simulink model "Citation"  (R2018a)
settings: Solver=ode5  StartTime=0.0  StopTime=500  FixedStep=0.01  RelTol=1e-3  EnableMultiTasking=on
InitFcn:
  | initcit
values from neighbouring files (symbols this model uses):
  aeroinit = [dp_ini;inicoef('CX0');inicoef('CXa');inicoef('CXa2');inicoef('CXq')     ;inicoef('CXde');inicoef('CY0');inicoef('CYB');inicoef('CYp');inicoef('CYr')     ;inicoef('CYda');inicoef('CYdr');inicoef('CZ0');inicoef('CZa');inicoef('CZq')     ;inicoef('CZde');inicoef('Cl0');inicoef('ClB');inicoef('Clp');inicoef('Clr')     ;inicoef('Clda');inicoef('Cldr');inicoef('Cm0');inicoef('Cma');inicoef('Cmq')     ; ...(+113 chars)    [initcit.m]
  h_l_old = zeros(6,sample_size)    [initcit.m]
  h_m_old = zeros(4,sample_size)    [initcit.m]
  h_n_old = zeros(6,sample_size)    [initcit.m]
  h_X_old = zeros(5,sample_size)    [initcit.m]
  h_Y_old = zeros(6,sample_size)    [initcit.m]
  h_Z_old = zeros(4,sample_size)    [initcit.m]
  I = [massinit(5),0, -massinit(8);0, massinit(6),0;-massinit(8),0, massinit(7)]    [initcit.m]
  p_l = [inicoef('Cl0');inicoef('ClB');inicoef('Clp');inicoef('Clr')     ;inicoef('Clda');inicoef('Cldr')].*ones(6,sample_size)    [initcit.m]
  p_m = [inicoef('Cm0');inicoef('Cma');inicoef('Cmq')     ;inicoef('Cmde')].*ones(4,sample_size)    [initcit.m]
  p_n = 0.71*ones(6,sample_size)    [initcit.m]
  p_X = [inicoef('CX0');inicoef('CXa');inicoef('CXa2');inicoef('CXq')     ;inicoef('CXde')].*ones(5,sample_size)    [initcit.m]
  p_Y = [inicoef('CY0');inicoef('CYB');inicoef('CYp');inicoef('CYr')     ;inicoef('CYda');inicoef('CYdr')].*ones(6,sample_size)    [initcit.m]
  p_Z = [inicoef('CZ0');inicoef('CZa');inicoef('CZq')     ;inicoef('CZde')].*ones(4,sample_size)    [initcit.m]
  Pcov_l = 10000*eye(6)    [initcit.m]
  Pcov_m = 10000*eye(4)    [initcit.m]
  Pcov_n = 10000*eye(6)    [initcit.m]
  Pcov_X = 10000*eye(5)    [initcit.m]
  Pcov_Y = 10000*eye(6)    [initcit.m]
  Pcov_Z = 10000*eye(4)    [initcit.m]
  T0 = 288.15    [rho_test.m]
  Vw915 = 0    [initcit.m]
  winddir = 45*(pi/180)    (= 0.785398163397)    [initcit.m]
  x0 = []    [cessnac550_3d_sfnc.m]    (also in sfunxyauto.m)
  y_l = zeros(1,sample_size)    [initcit.m]
  y_l_est_old = zeros(size(y_l))    [initcit.m]
  y_m = zeros(1,sample_size)    [initcit.m]
  y_m_est_old = zeros(size(y_m))    [initcit.m]
  y_n = zeros(1,sample_size)    [initcit.m]
  y_n_est_old = zeros(size(y_n))    [initcit.m]
  y_X = zeros(1,sample_size)    [initcit.m]
  y_X_est_old = zeros(size(y_X))    [initcit.m]
  y_Y = zeros(1,sample_size)    [initcit.m]
  y_Y_est_old = zeros(size(y_Y))    [initcit.m]
  y_Z = zeros(1,sample_size)    [initcit.m]
  y_Z_est_old = zeros(size(y_Z))    [initcit.m]
undefined symbols (not defined in the file or in its folder): chord, cv1, cv2, cv3, cv4, deltagmax1, deltagmax2, deltagmax3, deltagmax4, Deng, ealphag, ealphas, g0, hDME, hGS, kt1, kt2, kt3, lh, massinit, matbuaf, matdaf, matdam, matdbbf, matdeaf, matdgaf, matdqaf, matduaf, matdwaw, matedhr, mateif, matelhr, matemhr, matemv1, matemv2, matemve, matetam, mateuaf, matfaaf, matfaxl, matff, matibaf, matibb, matibmh, matipaf, matipmh, matiraf, matiuaf, matiwaf, matlaf, matlam, matleaf, matleam, matlgaf, matlqaf, matluaf, matmaaf, matmaam, matmaf, matmam ... (+75)
libraries: simulink x5, templibrary x3, vrlib x1
(part 6 of 6)

== matlab function Citation/Aerodynamic Parameter Estimation/CZ/MATLAB Function ==
  data: P_cov input; P_cov output; pk input; y_new input; hk_new input; y_old input; y_est_old input; h_old input; counter input; pk output; y_old output; y_est_old output; h_old output; forget input; counter output; y_est output; y_new output
function [P_cov, pk,y_old,y_est_old,h_old,counter,y_est,y_new] ...
    =LSQ(P_cov,pk,y_new,hk_new,y_old,y_est_old,h_old,counter,forget)
    lambda=forget;
    P=P_cov;
    p=pk(:,1);
    h=hk_new;
    y=y_new;
    Lk=P*h*(1/(h'*P*h+lambda));
    P=(eye(length(P))-Lk*h')*P*(1/lambda);
    
    p=p+Lk*(y-h'*p);   
    P_cov=P;   
    y_est=h'*p;
 
    
    %% Shift value history
    pk=shift(pk,p);
    y_est_old=(shift(y_est_old',y_est'))'; %this array is oriented vertically 
    h_old=shift(h_old,h);
    y_old=(shift(y_old',y_new'))';          %this array is oriented vertically 
    
    
    
    
    %shift array content right and insert new entry 
   
    function array = shift(array,insert)  

        for i=1:(size(array,2)-1)
             j=size(array,2)-i+1;
               array(:,j)=array(:,j-1);
        end
        array(:,1)=insert(:);

    end
%%
counter=counter+1;
end

== matlab function Citation/Aerodynamic Parameter Estimation/Cl/MATLAB Function ==
  data: P_cov input; P_cov output; pk input; y_new input; hk_new input; y_old input; y_est_old input; h_old input; counter input; pk output; y_old output; y_est_old output; h_old output; forget input; counter output; y_est output; y_new output
function [P_cov, pk,y_old,y_est_old,h_old,counter,y_est,y_new] ...
    =LSQ(P_cov,pk,y_new,hk_new,y_old,y_est_old,h_old,counter,forget)
    lambda=forget;
    P=P_cov;
    p=pk(:,1);
    h=hk_new;
    y=y_new;
    Lk=P*h*(1/(h'*P*h+lambda));
    P=(eye(length(P))-Lk*h')*P*(1/lambda);
    
    p=p+Lk*(y-h'*p);   
    P_cov=P;   
    y_est=h'*p;
 
    
    %% Shift value history
    pk=shift(pk,p);
    y_est_old=(shift(y_est_old',y_est'))'; %this array is oriented vertically 
    h_old=shift(h_old,h);
    y_old=(shift(y_old',y_new'))';          %this array is oriented vertically 
    
    
    
    
    %shift array content right and insert new entry 
   
    function array = shift(array,insert)  

        for i=1:(size(array,2)-1)
             j=size(array,2)-i+1;
               array(:,j)=array(:,j-1);
        end
        array(:,1)=insert(:);

    end
%%
counter=counter+1;
end

== matlab function Citation/Aerodynamic Parameter Estimation/Cm/MATLAB Function ==
  data: P_cov input; P_cov output; pk input; y_new input; hk_new input; y_old input; y_est_old input; h_old input; counter input; pk output; y_old output; y_est_old output; h_old output; forget input; counter output; y_est output; y_new output
function [P_cov, pk,y_old,y_est_old,h_old,counter,y_est,y_new] ...
    =LSQ(P_cov,pk,y_new,hk_new,y_old,y_est_old,h_old,counter,forget)
    lambda=forget;
    P=P_cov;
    p=pk(:,1);
    h=hk_new;
    y=y_new;
    Lk=P*h*(1/(h'*P*h+lambda));
    P=(eye(length(P))-Lk*h')*P*(1/lambda);
    
    p=p+Lk*(y-h'*p);   
    P_cov=P;   
    y_est=h'*p;
 
    
    %% Shift value history
    pk=shift(pk,p);
    y_est_old=(shift(y_est_old',y_est'))'; %this array is oriented vertically 
    h_old=shift(h_old,h);
    y_old=(shift(y_old',y_new'))';          %this array is oriented vertically 
    
    
    
    
    %shift array content right and insert new entry 
   
    function array = shift(array,insert)  

        for i=1:(size(array,2)-1)
             j=size(array,2)-i+1;
               array(:,j)=array(:,j-1);
        end
        array(:,1)=insert(:);

    end
%%
counter=counter+1;
end

== matlab function Citation/Aerodynamic Parameter Estimation/Cn/MATLAB Function ==
  data: P_cov input; P_cov output; pk input; y_new input; hk_new input; y_old input; y_est_old input; h_old input; counter input; pk output; y_old output; y_est_old output; h_old output; forget input; counter output; y_est output; y_new output
function [P_cov, pk,y_old,y_est_old,h_old,counter,y_est,y_new] ...
    =LSQ(P_cov,pk,y_new,hk_new,y_old,y_est_old,h_old,counter,forget)
    lambda=forget;
    P=P_cov;
    p=pk(:,1);
    h=hk_new;
    y=y_new;
    Lk=P*h*(1/(h'*P*h+lambda));
    P=(eye(length(P))-Lk*h')*P*(1/lambda);
    
    p=p+Lk*(y-h'*p);   
    P_cov=P;   
    y_est=h'*p;
 
    
    %% Shift value history
    pk=shift(pk,p);
    y_est_old=(shift(y_est_old',y_est'))'; %this array is oriented vertically 
    h_old=shift(h_old,h);
    y_old=(shift(y_old',y_new'))';          %this array is oriented vertically 
    
    
    
    
    %shift array content right and insert new entry 
   
    function array = shift(array,insert)  

        for i=1:(size(array,2)-1)
             j=size(array,2)-i+1;
               array(:,j)=array(:,j-1);
        end
        array(:,1)=insert(:);

    end
%%
counter=counter+1;
end

== matlab function Citation/Cessna Citation 500/Controllers/NDI rotational rate controller/b^-1 ==
  data: ve input; delta output; aerodat input; I parameter; chord parameter; span parameter; S parameter; mat_old output; mat_old input
function [delta, mat_old]  = fcn(ve,aerodat, I, chord, span, S,mat_old)
dp=aerodat(1); %dynamic pressure =0.5*rho*V^2*S
clda=aerodat(21);
cldr=aerodat(22);
cmde=aerodat(26);
cnda=aerodat(31);
cndr=aerodat(32);
mat=[span*clda, 0, span*cldr;
    0, chord*cmde, 0;
    span*cnda, 0, span*cndr];

if det(mat)==0 %take an older matrix if it is non-invertible
   mat=mat_old; 
else
    mat_old=mat;
end
amat=mat^(-1)*I;
delta=amat*(1/(dp))*ve;
dummy=1;

== matlab function Citation/Cessna Citation 500/Controllers/NDI rotational rate controller/a ==
  data: aerodat input; state input; y output; I parameter; span parameter; chord parameter
function y = fcn(aerodat,state, I, span, chord)
dp=aerodat(1);
p=state(1);
q=state(2);
r=state(3);
b=span;
c=chord;
V=state(4);
alpha=state(5);
beta=state(6);
Cl=aerodat(17:22);
Cm=aerodat(23:26);
Cn=aerodat(27:32);


Cla=Cl(1)+Cl(2)*beta+(Cl(3)*(p*b)/(2*V))+(Cl(4)*(r*b/(2*V)));
Cma=Cm(1)+Cm(2)*alpha+(Cm(3)*(q*c)/(2*V));
Cna=Cn(1)+Cn(2)*beta+(Cn(3)*(p*b)/(2*V))+(Cn(4)*(r*b/(2*V)));
term1=cross(state(1:3),I*state(1:3));
term2=dp*[b*Cla; c*Cma; b*Cna];
term3=term1-term2;
y=-1*(I^(-1)*term3);

== matlab function Citation/Aerodynamic Parameter Estimation/Statistics 2/Auto_correlation/autocorrelation ==
  data: delta input; PI_kgap output; kgap input; kgap_avg input; counter input; kgap_avg output; counter output
function [PI_kgap,kgap_avg,counter] = fcn(delta,kgap,kgap_avg,counter)

PI_kgap=(delta(1)*delta(1+kgap));
if counter>=1
    kgap_avg=kgap_avg+(PI_kgap/counter);
else
    kgap_avg=PI_kgap;
end

counter=counter+1;
end

== matlab function Citation/Aerodynamic Parameter Estimation/Statistics 2/moving average square ==
  data: delta input; av output
function av = fcn(delta)
av=0;
nav=length(delta);
k=nav;
for i=0:(nav-1)
    av=av+(delta(k-i))^2;
end
av=av/k;
end

== matlab function Citation/Aerodynamic Parameter Estimation/Statistics 2/variance/MATLAB Function ==
  data: delta input; var output; delta_avg input; counter input; delta_avg output; counter output; sigma_avg input; sigma_avg output
function [var,delta_avg,counter,sigma_avg] = variance(delta,delta_avg,counter,sigma_avg)

if counter >=1
    delta_avg=delta_avg+delta/counter;
    var=0;
    if counter >=2
        var=((delta-delta_avg)^2);
        
        s=sigma_avg(1)+sqrt(var)/(counter-1);
        sigma_avg=[s;-s];
    end
else
    delta_avg=delta;
    var=0;
end



counter=counter+1;

== matlab function Citation/Aerodynamic Parameter Estimation/Statistics 3/Auto_correlation/autocorrelation ==
  data: delta input; PI_kgap output; kgap input; kgap_avg input; counter input; kgap_avg output; counter output
function [PI_kgap,kgap_avg,counter] = fcn(delta,kgap,kgap_avg,counter)

PI_kgap=(delta(1)*delta(1+kgap));
if counter>=1
    kgap_avg=kgap_avg+(PI_kgap/counter);
else
    kgap_avg=PI_kgap;
end

counter=counter+1;
end

== matlab function Citation/Aerodynamic Parameter Estimation/Statistics 3/moving average square ==
  data: delta input; av output
function av = fcn(delta)
av=0;
nav=length(delta);
k=nav;
for i=0:(nav-1)
    av=av+(delta(k-i))^2;
end
av=av/k;
end

== matlab function Citation/Aerodynamic Parameter Estimation/Statistics 3/variance/MATLAB Function ==
  data: delta input; var output; delta_avg input; counter input; delta_avg output; counter output; sigma_avg input; sigma_avg output
function [var,delta_avg,counter,sigma_avg] = variance(delta,delta_avg,counter,sigma_avg)

if counter >=1
    delta_avg=delta_avg+delta/counter;
    var=0;
    if counter >=2
        var=((delta-delta_avg)^2);
        
        s=sigma_avg(1)+(sqrt(var)/(counter-1));
        sigma_avg=[s;-s];
    end
else
    delta_avg=delta;
    var=0;
end



counter=counter+1;

== matlab function Citation/Aerodynamic Parameter Estimation/Statistics 4/Auto_correlation/autocorrelation ==
  data: delta input; PI_kgap output; kgap input; kgap_avg input; counter input; kgap_avg output; counter output
function [PI_kgap,kgap_avg,counter] = fcn(delta,kgap,kgap_avg,counter)

PI_kgap=(delta(1)*delta(1+kgap));
if counter>=1
    kgap_avg=kgap_avg+(PI_kgap/counter);
else
    kgap_avg=PI_kgap;
end

counter=counter+1;
end

== matlab function Citation/Aerodynamic Parameter Estimation/Statistics 4/moving average square ==
  data: delta input; av output
function av = fcn(delta)
av=0;
nav=length(delta);
k=nav;
for i=0:(nav-1)
    av=av+(delta(k-i))^2;
end
av=av/k;
end

== matlab function Citation/Aerodynamic Parameter Estimation/Statistics 4/variance/MATLAB Function ==
  data: delta input; var output; delta_avg input; counter input; delta_avg output; counter output; sigma_avg input; sigma_avg output
function [var,delta_avg,counter,sigma_avg] = variance(delta,delta_avg,counter,sigma_avg)

if counter >=1
    delta_avg=delta_avg+delta/counter;
    var=0;
    if counter >=2
        var=((delta-delta_avg)^2);
        
        s=sigma_avg(1)+sqrt(var)/(counter-1);
        sigma_avg=[s;-s];
    end
else
    delta_avg=delta;
    var=0;
end



counter=counter+1;
